simulink model "Manu6DOF_MICO_NE_v6articulation2019b"  (R2019b)
settings: Solver=ode5  StartTime=0.0  StopTime=10.0  FixedStep=0.001  RelTol=1e-3
undefined symbols (not defined in the file): f, Sub02MIHM
libraries: instrumentlib x27, dspnetwork x24, simulink x7, dspmtrx3 x3, dspsrcs4 x1
(part 1 of 3)
settings Model: Creator=nisit  LastModifiedBy=Jskyl

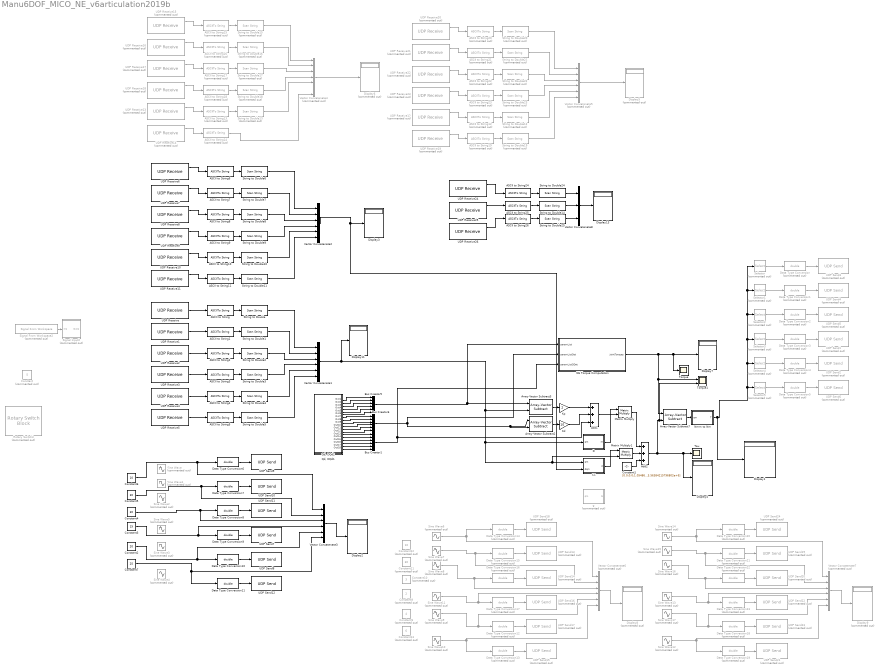
== system Manu6DOF_MICO_NE_v6articulation2019b ==
  ASCII to String{,1..11,24..26} (15 alike) : ASCIIToString
  ASCII to String{12..23} (12 alike) : ASCIIToString  Commented=on
  Add1 : Sum  Inputs=+++
  Add2 : Sum  Inputs=+++
  Array-Vector Subtract2 : dspmtrx3/Array-Vector Subtract  Dimension=1  V_Source=Input port  V_VectFromMask=[0.5 0.25]  prodOutputSignedness=Auto  roundingMode=Floor  overflowMode=off  firstCoeffSignedness=Auto  firstCoeffDataTypeStr=Inherit: Same word length as input  firstCoeffMin=[]  firstCoeffMax=[]  firstCoeffLastDataTypeStr=Inherit: Same word length as input  accumSignedness=Auto  outputSignedness=Auto  outputDataTypeStr=Inherit: Same as accumulator  outputMin=[]  outputMax=[]  outputLastDataTypeStr=Inherit: Same as accumulator
      settings: SourceProductBaseCode=DS
  Array-Vector Subtract3 : dspmtrx3/Array-Vector Subtract  Dimension=1  V_Source=Input port  V_VectFromMask=[0.5 0.25]  prodOutputSignedness=Auto  roundingMode=Floor  overflowMode=off  firstCoeffSignedness=Auto  firstCoeffDataTypeStr=Inherit: Same word length as input  firstCoeffMin=[]  firstCoeffMax=[]  firstCoeffLastDataTypeStr=Inherit: Same word length as input  accumSignedness=Auto  outputSignedness=Auto  outputDataTypeStr=Inherit: Same as accumulator  outputMin=[]  outputMax=[]  outputLastDataTypeStr=Inherit: Same as accumulator
      settings: SourceProductBaseCode=DS
  Array-Vector Subtract7 : dspmtrx3/Array-Vector Subtract  Dimension=1  V_Source=Input port  V_VectFromMask=[0.5 0.25]  prodOutputSignedness=Auto  roundingMode=Floor  overflowMode=off  firstCoeffSignedness=Auto  firstCoeffDataTypeStr=Inherit: Same word length as input  firstCoeffMin=[]  firstCoeffMax=[]  firstCoeffLastDataTypeStr=Inherit: Same word length as input  accumSignedness=Auto  outputSignedness=Auto  outputDataTypeStr=Inherit: Same as accumulator  outputMin=[]  outputMax=[]  outputLastDataTypeStr=Inherit: Same as accumulator
      settings: SourceProductBaseCode=DS
  Bus Creator1 : BusCreator  Inputs=6
  Bus Creator5 : BusCreator  Inputs=6
  Bus Creator6 : BusCreator  Inputs=6
  C1 : MATLAB Function  TreatAsAtomicUnit=on
  Constant : Constant  Commented=on  Value=5
  Constant1 : Constant  Value=[0.0;0.0;1.054861899110132e+7;sqrt(3.0).*2.596216141849145e-10+4.239942722516781e+6;sqrt(3.0).*2.389220043780056e-10-3.901892440242401e+6;sqrt(3.0).*(-6.546671837132898e-10)+3.56384215796802e+6]
  Constant10 : Constant  Commented=on  Value=3
  Constant11 : Constant  Commented=on  Value=30
  Constant12 : Constant  Commented=on  Value=10
  Constant13 : Constant  Commented=on  Value=6
  Constant2 : Constant  Value=20
  Constant3 : Constant  Value=15
  Constant4 : Constant  Value=30
  Constant5 : Constant  Value=30
  Constant6 : Constant  Value=10
  Constant7 : Constant  Value=25
  Constant8 : Constant  Commented=on  Value=4
  Constant9 : Constant  Commented=on  Value=2
  D : MATLAB Function  TreatAsAtomicUnit=on
  Data Type Conversion{,1..5,12..23} (18 alike) : DataTypeConversion  Commented=on  OutDataTypeStr=double  ConvertRealWorld=Stored Integer (SI)
  Data Type Conversion{6..11} (6 alike) : DataTypeConversion  OutDataTypeStr=double  ConvertRealWorld=Stored Integer (SI)
  Display{1..4,7,11,13} (7 alike) : Display
  Display{5..6,8..9} (4 alike) : Display  Commented=on
  Kd : Gain  Gain=10
  Kp : Gain  Gain=2
  Matrix Multiply : Product  Multiplication=Matrix(*)
  Matrix Multiply1 : Product  Multiplication=Matrix(*)
  NE Torque Computation : MATLAB Function  TreatAsAtomicUnit=on
  Nmm to Nm : MATLAB Function  TreatAsAtomicUnit=on
  "Qd, DQd1" : Subsystem
  "Qd, DQd2" : Subsystem
  Rotary Switch3 : RotarySwitchBlock  Commented=on
      settings: Values={{'Left', 'Right', 'Out', 'In', 'Up', 'Down'}, [1 4 2 5 3 6]}
  Selector : Selector  Commented=on  InputPortWidth=6  IndexOptions=Index vector (dialog)  Indices=[1]  OutputSizes=1
  Selector1 : Selector  Commented=on  InputPortWidth=6  IndexOptions=Index vector (dialog)  Indices=[2]  OutputSizes=1
  Selector2 : Selector  Commented=on  InputPortWidth=6  IndexOptions=Index vector (dialog)  Indices=[3]  OutputSizes=1
  Selector3 : Selector  Commented=on  InputPortWidth=6  IndexOptions=Index vector (dialog)  Indices=[4]  OutputSizes=1
  Selector4 : Selector  Commented=on  InputPortWidth=6  IndexOptions=Index vector (dialog)  Indices=[5]  OutputSizes=1
  Selector5 : Selector  Commented=on  InputPortWidth=6  IndexOptions=Index vector (dialog)  Indices=[6]  OutputSizes=1
  Signal From Workspace2 : dspsrcs4/Signal From Workspace  Commented=on  X=transpose(Sub02MIHM)  Ts=0.004  nsamps=1  OutputAfterFinalValue=Setting to zero  ignoreOrWarnInputAndFrameLengths=off  OutputFrames=off
  Signal Input2 : Subsystem  Commented=on
  Sine Wave : Sin  Commented=on  Amplitude=25  Frequency=15  SampleTime=0
  Sine Wave1 : Sin  Commented=on  Amplitude=30  Frequency=5  SampleTime=0
  Sine Wave10 : Sin  Commented=on  Amplitude=7  Frequency=8  SampleTime=0
  Sine Wave11 : Sin  Commented=on  Amplitude=9  Frequency=3  SampleTime=0
  Sine Wave12 : Sin  Commented=on  Amplitude=7  Frequency=8  SampleTime=0
  Sine Wave13 : Sin  Commented=on  Amplitude=9  Frequency=3  SampleTime=0
  Sine Wave14 : Sin  Commented=on  Amplitude=25  Frequency=15  SampleTime=0
  Sine Wave15 : Sin  Commented=on  Amplitude=30  Frequency=5  SampleTime=0
  Sine Wave16 : Sin  Commented=on  Amplitude=102  SampleTime=0
  Sine Wave17 : Sin  Commented=on  Amplitude=10  Frequency=15  SampleTime=0
  Sine Wave2 : Sin  Commented=on  Amplitude=102  SampleTime=0
  Sine Wave3 : Sin  Commented=on  Amplitude=10  Frequency=15  SampleTime=0
  Sine Wave4 : Sin  Commented=on  Amplitude=7  Frequency=8  SampleTime=0
  Sine Wave5 : Sin  Commented=on  Amplitude=9  Frequency=3  SampleTime=0
  Sine Wave6 : Sin  Commented=on  Amplitude=25  Frequency=15  SampleTime=0
  Sine Wave7 : Sin  Commented=on  Amplitude=30  Frequency=5  SampleTime=0
  Sine Wave8 : Sin  Commented=on  Amplitude=102  SampleTime=0
  Sine Wave9 : Sin  Commented=on  Amplitude=10  Frequency=15  SampleTime=0
  String to Double{,1..11,14,24..25} (15 alike) : ScanString  Format="\"%lf\""
  String to Double{12..13,15..23} (11 alike) : ScanString  Commented=on  Format="\"%lf\""
  Tau : Scope
  Torque : Scope
  Torque1 : Scope  NumInputPorts=2
  UDP Receive : instrumentlib/UDP Receive  Host=localhost  Port=2001  LocalPort=2001  EnablePortSharing=off  GetLatestData=off  DataSize="[5  1]"  DataType=uint8  ASCIIFormatting=%f,  Terminator=LF  ByteOrder=BigEndian  EnableBlockingMode=on  Timeout=10  SampleTime=0.01  LocalAddress=127.0.0.1
  UDP Receive1 : instrumentlib/UDP Receive  Host=localhost  Port=2002  LocalPort=2002  EnablePortSharing=off  GetLatestData=off  DataSize="[5  1]"  DataType=uint8  ASCIIFormatting=%f,  Terminator=LF  ByteOrder=BigEndian  EnableBlockingMode=on  Timeout=10  SampleTime=0.01  LocalAddress=127.0.0.1
  UDP Receive10 : instrumentlib/UDP Receive  Host=localhost  Port=4005  LocalPort=4005  EnablePortSharing=off  GetLatestData=off  DataSize="[5  1]"  DataType=uint8  ASCIIFormatting=%f,  Terminator=LF  ByteOrder=BigEndian  EnableBlockingMode=off  Timeout=10  SampleTime=0.01  LocalAddress=127.0.0.1
  UDP Receive11 : instrumentlib/UDP Receive  Host=localhost  Port=4006  LocalPort=4006  EnablePortSharing=off  GetLatestData=off  DataSize="[5  1]"  DataType=uint8  ASCIIFormatting=%f,  Terminator=LF  ByteOrder=BigEndian  EnableBlockingMode=off  Timeout=10  SampleTime=0.01  LocalAddress=127.0.0.1
  UDP Receive12 : instrumentlib/UDP Receive  Commented=on  Host=localhost  Port=7005  LocalPort=7005  EnablePortSharing=off  GetLatestData=off  DataSize="[5  1]"  DataType=uint8  ASCIIFormatting=%f,  Terminator=LF  ByteOrder=BigEndian  EnableBlockingMode=off  Timeout=10  SampleTime=0.01  LocalAddress=127.0.0.1
  UDP Receive13 : instrumentlib/UDP Receive  Commented=on  Host=localhost  Port=6005  LocalPort=6005  EnablePortSharing=off  GetLatestData=off  DataSize="[5  1]"  DataType=uint8  ASCIIFormatting=%f,  Terminator=LF  ByteOrder=BigEndian  EnableBlockingMode=off  Timeout=10  SampleTime=0.01  LocalAddress=127.0.0.1
  UDP Receive14 : instrumentlib/UDP Receive  Commented=on  Host=localhost  Port=6006  LocalPort=6006  EnablePortSharing=off  GetLatestData=off  DataSize="[5  1]"  DataType=uint8  ASCIIFormatting=%f,  Terminator=LF  ByteOrder=BigEndian  EnableBlockingMode=off  Timeout=10  SampleTime=0.01  LocalAddress=127.0.0.1
  UDP Receive15 : instrumentlib/UDP Receive  Commented=on  Host=localhost  Port=6001  LocalPort=6001  EnablePortSharing=off  GetLatestData=off  DataSize="[5  1]"  DataType=uint8  ASCIIFormatting=%f,  Terminator=LF  ByteOrder=BigEndian  EnableBlockingMode=off  Timeout=10  SampleTime=0.01  LocalAddress=127.0.0.1
  UDP Receive16 : instrumentlib/UDP Receive  Commented=on  Host=localhost  Port=6002  LocalPort=6002  EnablePortSharing=off  GetLatestData=off  DataSize="[5  1]"  DataType=uint8  ASCIIFormatting=%f,  Terminator=LF  ByteOrder=BigEndian  EnableBlockingMode=off  Timeout=10  SampleTime=0.01  LocalAddress=127.0.0.1
  UDP Receive17 : instrumentlib/UDP Receive  Commented=on  Host=localhost  Port=6003  LocalPort=6003  EnablePortSharing=off  GetLatestData=off  DataSize="[5  1]"  DataType=uint8  ASCIIFormatting=%f,  Terminator=LF  ByteOrder=BigEndian  EnableBlockingMode=off  Timeout=10  SampleTime=0.01  LocalAddress=127.0.0.1
  UDP Receive18 : instrumentlib/UDP Receive  Commented=on  Host=localhost  Port=6004  LocalPort=6004  EnablePortSharing=off  GetLatestData=off  DataSize="[5  1]"  DataType=uint8  ASCIIFormatting=%f,  Terminator=LF  ByteOrder=BigEndian  EnableBlockingMode=off  Timeout=10  SampleTime=0.01  LocalAddress=127.0.0.1
  UDP Receive19 : instrumentlib/UDP Receive  Commented=on  Host=localhost  Port=7006  LocalPort=7006  EnablePortSharing=off  GetLatestData=off  DataSize="[5  1]"  DataType=uint8  ASCIIFormatting=%f,  Terminator=LF  ByteOrder=BigEndian  EnableBlockingMode=off  Timeout=10  SampleTime=0.01  LocalAddress=127.0.0.1
  UDP Receive2 : instrumentlib/UDP Receive  Host=localhost  Port=2003  LocalPort=2003  EnablePortSharing=off  GetLatestData=off  DataSize="[5  1]"  DataType=uint8  ASCIIFormatting=%f,  Terminator=LF  ByteOrder=BigEndian  EnableBlockingMode=on  Timeout=10  SampleTime=0.01  LocalAddress=127.0.0.1
  UDP Receive20 : instrumentlib/UDP Receive  Commented=on  Host=localhost  Port=7001  LocalPort=7001  EnablePortSharing=off  GetLatestData=off  DataSize="[5  1]"  DataType=uint8  ASCIIFormatting=%f,  Terminator=LF  ByteOrder=BigEndian  EnableBlockingMode=off  Timeout=10  SampleTime=0.01  LocalAddress=127.0.0.1
  UDP Receive21 : instrumentlib/UDP Receive  Commented=on  Host=localhost  Port=7002  LocalPort=7002  EnablePortSharing=off  GetLatestData=off  DataSize="[5  1]"  DataType=uint8  ASCIIFormatting=%f,  Terminator=LF  ByteOrder=BigEndian  EnableBlockingMode=off  Timeout=10  SampleTime=0.01  LocalAddress=127.0.0.1
  UDP Receive22 : instrumentlib/UDP Receive  Commented=on  Host=localhost  Port=7003  LocalPort=7003  EnablePortSharing=off  GetLatestData=off  DataSize="[5  1]"  DataType=uint8  ASCIIFormatting=%f,  Terminator=LF  ByteOrder=BigEndian  EnableBlockingMode=off  Timeout=10  SampleTime=0.01  LocalAddress=127.0.0.1
  UDP Receive23 : instrumentlib/UDP Receive  Commented=on  Host=localhost  Port=7004  LocalPort=7004  EnablePortSharing=off  GetLatestData=off  DataSize="[5  1]"  DataType=uint8  ASCIIFormatting=%f,  Terminator=LF  ByteOrder=BigEndian  EnableBlockingMode=off  Timeout=10  SampleTime=0.01  LocalAddress=127.0.0.1
  UDP Receive24 : instrumentlib/UDP Receive  Host=localhost  Port=5100  LocalPort=5100  EnablePortSharing=off  GetLatestData=off  DataSize="[5  1]"  DataType=uint8  ASCIIFormatting=%f,  Terminator=LF  ByteOrder=BigEndian  EnableBlockingMode=off  Timeout=10  SampleTime=0.01  LocalAddress=127.0.0.1
  UDP Receive25 : instrumentlib/UDP Receive  Host=localhost  Port=5200  LocalPort=5200  EnablePortSharing=off  GetLatestData=off  DataSize="[5  1]"  DataType=uint8  ASCIIFormatting=%f,  Terminator=LF  ByteOrder=BigEndian  EnableBlockingMode=off  Timeout=10  SampleTime=0.01  LocalAddress=127.0.0.1
  UDP Receive26 : instrumentlib/UDP Receive  Host=localhost  Port=5300  LocalPort=5300  EnablePortSharing=off  GetLatestData=off  DataSize="[5  1]"  DataType=uint8  ASCIIFormatting=%f,  Terminator=LF  ByteOrder=BigEndian  EnableBlockingMode=off  Timeout=10  SampleTime=0.01  LocalAddress=127.0.0.1
  UDP Receive3 : instrumentlib/UDP Receive  Host=localhost  Port=2004  LocalPort=2004  EnablePortSharing=off  GetLatestData=off  DataSize="[5  1]"  DataType=uint8  ASCIIFormatting=%f,  Terminator=LF  ByteOrder=BigEndian  EnableBlockingMode=on  Timeout=10  SampleTime=0.01  LocalAddress=127.0.0.1
  UDP Receive4 : instrumentlib/UDP Receive  Host=localhost  Port=2005  LocalPort=2005  EnablePortSharing=off  GetLatestData=off  DataSize="[5  1]"  DataType=uint8  ASCIIFormatting=%f,  Terminator=LF  ByteOrder=BigEndian  EnableBlockingMode=on  Timeout=10  SampleTime=0.01  LocalAddress=127.0.0.1
  UDP Receive5 : instrumentlib/UDP Receive  Host=localhost  Port=2006  LocalPort=2006  EnablePortSharing=off  GetLatestData=off  DataSize="[5  1]"  DataType=uint8  ASCIIFormatting=%f,  Terminator=LF  ByteOrder=BigEndian  EnableBlockingMode=on  Timeout=10  SampleTime=0.01  LocalAddress=127.0.0.1
  UDP Receive6 : instrumentlib/UDP Receive  Host=localhost  Port=4001  LocalPort=4001  EnablePortSharing=off  GetLatestData=off  DataSize="[5  1]"  DataType=uint8  ASCIIFormatting=%f,  Terminator=LF  ByteOrder=BigEndian  EnableBlockingMode=off  Timeout=10  SampleTime=0.01  LocalAddress=127.0.0.1
  UDP Receive7 : instrumentlib/UDP Receive  Host=localhost  Port=4002  LocalPort=4002  EnablePortSharing=off  GetLatestData=off  DataSize="[5  1]"  DataType=uint8  ASCIIFormatting=%f,  Terminator=LF  ByteOrder=BigEndian  EnableBlockingMode=off  Timeout=10  SampleTime=0.01  LocalAddress=127.0.0.1
  UDP Receive8 : instrumentlib/UDP Receive  Host=localhost  Port=4003  LocalPort=4003  EnablePortSharing=off  GetLatestData=off  DataSize="[5  1]"  DataType=uint8  ASCIIFormatting=%f,  Terminator=LF  ByteOrder=BigEndian  EnableBlockingMode=off  Timeout=10  SampleTime=0.01  LocalAddress=127.0.0.1
  UDP Receive9 : instrumentlib/UDP Receive  Host=localhost  Port=4004  LocalPort=4004  EnablePortSharing=off  GetLatestData=off  DataSize="[5  1]"  DataType=uint8  ASCIIFormatting=%f,  Terminator=LF  ByteOrder=BigEndian  EnableBlockingMode=off  Timeout=10  SampleTime=0.01  LocalAddress=127.0.0.1
  UDP Send1 : dspnetwork/UDP Send  Commented=on  remoteURL='127.0.0.1'  remotePort=3004  localURL='0.0.0.0'  localPortSource=Automatically determine  localPort=-1  sampletime=-1  blockPlatform=[]  separateLengthPort=0
  UDP Send10 : dspnetwork/UDP Send  remoteURL='127.0.0.1'  remotePort=5002  localURL='0.0.0.0'  localPortSource=Automatically determine  localPort=-1  sampletime=-1  blockPlatform=[]  separateLengthPort=0
  UDP Send11 : dspnetwork/UDP Send  remoteURL='127.0.0.1'  remotePort=5003  localURL='0.0.0.0'  localPortSource=Automatically determine  localPort=-1  sampletime=-1  blockPlatform=[]  separateLengthPort=0
  UDP Send12 : dspnetwork/UDP Send  remoteURL='127.0.0.1'  remotePort=5006  localURL='0.0.0.0'  localPortSource=Automatically determine  localPort=-1  sampletime=-1  blockPlatform=[]  separateLengthPort=0
  UDP Send13 : dspnetwork/UDP Send  Commented=on  remoteURL='127.0.0.1'  remotePort=8002  localURL='0.0.0.0'  localPortSource=Automatically determine  localPort=-1  sampletime=-1  blockPlatform=[]  separateLengthPort=0
  UDP Send14 : dspnetwork/UDP Send  Commented=on  remoteURL='127.0.0.1'  remotePort=8003  localURL='0.0.0.0'  localPortSource=Automatically determine  localPort=-1  sampletime=-1  blockPlatform=[]  separateLengthPort=0
  UDP Send15 : dspnetwork/UDP Send  Commented=on  remoteURL='127.0.0.1'  remotePort=8006  localURL='0.0.0.0'  localPortSource=Automatically determine  localPort=-1  sampletime=-1  blockPlatform=[]  separateLengthPort=0
  UDP Send16 : dspnetwork/UDP Send  Commented=on  remoteURL='127.0.0.1'  remotePort=8004  localURL='0.0.0.0'  localPortSource=Automatically determine  localPort=-1  sampletime=-1  blockPlatform=[]  separateLengthPort=0
  UDP Send17 : dspnetwork/UDP Send  Commented=on  remoteURL='127.0.0.1'  remotePort=8005  localURL='0.0.0.0'  localPortSource=Automatically determine  localPort=-1  sampletime=-1  blockPlatform=[]  separateLengthPort=0
  UDP Send18 : dspnetwork/UDP Send  Commented=on  remoteURL='127.0.0.1'  remotePort=8001  localURL='0.0.0.0'  localPortSource=Automatically determine  localPort=-1  sampletime=-1  blockPlatform=[]  separateLengthPort=0
  UDP Send19 : dspnetwork/UDP Send  Commented=on  remoteURL='127.0.0.1'  remotePort=9002  localURL='0.0.0.0'  localPortSource=Automatically determine  localPort=-1  sampletime=-1  blockPlatform=[]  separateLengthPort=0
  UDP Send2 : dspnetwork/UDP Send  Commented=on  remoteURL='127.0.0.1'  remotePort=3005  localURL='0.0.0.0'  localPortSource=Automatically determine  localPort=-1  sampletime=-1  blockPlatform=[]  separateLengthPort=0
  UDP Send20 : dspnetwork/UDP Send  Commented=on  remoteURL='127.0.0.1'  remotePort=9003  localURL='0.0.0.0'  localPortSource=Automatically determine  localPort=-1  sampletime=-1  blockPlatform=[]  separateLengthPort=0
  UDP Send21 : dspnetwork/UDP Send  Commented=on  remoteURL='127.0.0.1'  remotePort=9006  localURL='0.0.0.0'  localPortSource=Automatically determine  localPort=-1  sampletime=-1  blockPlatform=[]  separateLengthPort=0
  UDP Send22 : dspnetwork/UDP Send  Commented=on  remoteURL='127.0.0.1'  remotePort=9004  localURL='0.0.0.0'  localPortSource=Automatically determine  localPort=-1  sampletime=-1  blockPlatform=[]  separateLengthPort=0
  UDP Send23 : dspnetwork/UDP Send  Commented=on  remoteURL='127.0.0.1'  remotePort=9005  localURL='0.0.0.0'  localPortSource=Automatically determine  localPort=-1  sampletime=-1  blockPlatform=[]  separateLengthPort=0
  UDP Send24 : dspnetwork/UDP Send  Commented=on  remoteURL='127.0.0.1'  remotePort=9001  localURL='0.0.0.0'  localPortSource=Automatically determine  localPort=-1  sampletime=-1  blockPlatform=[]  separateLengthPort=0
  UDP Send3 : dspnetwork/UDP Send  Commented=on  remoteURL='127.0.0.1'  remotePort=3001  localURL='0.0.0.0'  localPortSource=Automatically determine  localPort=-1  sampletime=-1  blockPlatform=[]  separateLengthPort=0
  UDP Send4 : dspnetwork/UDP Send  Commented=on  remoteURL='127.0.0.1'  remotePort=3002  localURL='0.0.0.0'  localPortSource=Automatically determine  localPort=-1  sampletime=-1  blockPlatform=[]  separateLengthPort=0
  UDP Send5 : dspnetwork/UDP Send  Commented=on  remoteURL='127.0.0.1'  remotePort=3003  localURL='0.0.0.0'  localPortSource=Automatically determine  localPort=-1  sampletime=-1  blockPlatform=[]  separateLengthPort=0
  UDP Send6 : dspnetwork/UDP Send  Commented=on  remoteURL='127.0.0.1'  remotePort=3006  localURL='0.0.0.0'  localPortSource=Automatically determine  localPort=-1  sampletime=-1  blockPlatform=[]  separateLengthPort=0
  UDP Send7 : dspnetwork/UDP Send  remoteURL='127.0.0.1'  remotePort=5004  localURL='0.0.0.0'  localPortSource=Automatically determine  localPort=-1  sampletime=-1  blockPlatform=[]  separateLengthPort=0
  UDP Send8 : dspnetwork/UDP Send  remoteURL='127.0.0.1'  remotePort=5005  localURL='0.0.0.0'  localPortSource=Automatically determine  localPort=-1  sampletime=-1  blockPlatform=[]  separateLengthPort=0
  UDP Send9 : dspnetwork/UDP Send  remoteURL='127.0.0.1'  remotePort=5001  localURL='0.0.0.0'  localPortSource=Automatically determine  localPort=-1  sampletime=-1  blockPlatform=[]  separateLengthPort=0
  Vector Concatenate1 : Concatenate  NumInputs=6
  Vector Concatenate2 : Concatenate  NumInputs=6
  Vector Concatenate3 : Concatenate  NumInputs=6
  Vector Concatenate4 : Concatenate  Commented=on  NumInputs=7
  Vector Concatenate5 : Concatenate  Commented=on  NumInputs=6
  Vector Concatenate6 : Concatenate  Commented=on  NumInputs=6
  Vector Concatenate7 : Concatenate  Commented=on  NumInputs=6
  Vector Concatenate8 : Concatenate  NumInputs=3
  g : MATLAB Function  Commented=on  TreatAsAtomicUnit=on
  wires:
  D/1(M) -> Matrix Multiply/1
  Matrix Multiply1/1 -> Add2/2
  Array-Vector Subtract3/1 -> Kp/1
  Array-Vector Subtract2/1 -> Kd/1
  Matrix Multiply/1 -> Add2/1
  Kd/1 -> Add1/2
  Add1/1 -> Matrix Multiply/2
  Kp/1 -> Add1/1
  C1/1(C) -> Matrix Multiply1/1
  Array-Vector Subtract7/1 -> Nmm to Nm/1(qm)
  Add2/1 -> Torque1/2, Array-Vector Subtract7/2, Display4/1, Tau/1
  Constant1/1 -> Add2/3
  "Qd, DQd1"/15(Out15) -> Bus Creator1/3
  "Qd, DQd1"/10(Out10) -> Bus Creator6/4
  "Qd, DQd1"/17(Out17) -> Bus Creator1/5
  "Qd, DQd1"/9(Out9) -> Bus Creator6/3
  "Qd, DQd1"/11(Out11) -> Bus Creator6/5
  "Qd, DQd1"/6(Out6) -> Bus Creator5/6
  "Qd, DQd1"/12(Out12) -> Bus Creator6/6
  "Qd, DQd1"/13(Out13) -> Bus Creator1/1
  "Qd, DQd1"/18(Out18) -> Bus Creator1/6
  "Qd, DQd1"/16(Out16) -> Bus Creator1/4
  "Qd, DQd1"/1(Out1) -> Bus Creator5/1
  "Qd, DQd1"/2(Out2) -> Bus Creator5/2
  "Qd, DQd1"/7(Out7) -> Bus Creator6/1
  "Qd, DQd1"/5(Out5) -> Bus Creator5/5
  "Qd, DQd1"/3(Out3) -> Bus Creator5/3
  "Qd, DQd1"/8(Out8) -> Bus Creator6/2
  "Qd, DQd1"/14(Out14) -> Bus Creator1/2
  "Qd, DQd1"/4(Out4) -> Bus Creator5/4
  Signal From Workspace2/1 -> Signal Input2/1(In1)
  Data Type Conversion2/1 -> UDP Send5/1
  Selector5/1 -> Data Type Conversion5/1
  Data Type Conversion5/1 -> UDP Send6/1
  Selector4/1 -> Data Type Conversion4/1
  Data Type Conversion3/1 -> UDP Send1/1
  Data Type Conversion1/1 -> UDP Send4/1
  Data Type Conversion4/1 -> UDP Send2/1
  Selector2/1 -> Data Type Conversion2/1
  Selector/1 -> Data Type Conversion/1
  Selector1/1 -> Data Type Conversion1/1
  Data Type Conversion/1 -> UDP Send3/1
  Selector3/1 -> Data Type Conversion3/1
  NE Torque Computation/1(jointTorques) -> Display7/1, Torque/1, Array-Vector Subtract7/1, Torque1/1
  String to Double4/1 -> Vector Concatenate1/5
  ASCII to String2/1 -> String to Double2/1
  String to Double/1 -> Vector Concatenate1/1
  ASCII to String4/1 -> String to Double4/1
  String to Double2/1 -> Vector Concatenate1/3
  ASCII to String3/1 -> String to Double3/1
  String to Double5/1 -> Vector Concatenate1/6
  String to Double1/1 -> Vector Concatenate1/2
  ASCII to String1/1 -> String to Double1/1
  UDP Receive2/1 -> ASCII to String2/1
  UDP Receive/1 -> ASCII to String/1
  ASCII to String5/1 -> String to Double5/1
  UDP Receive3/1 -> ASCII to String3/1
  UDP Receive1/1 -> ASCII to String1/1
  ASCII to String/1 -> String to Double/1
  UDP Receive5/1 -> ASCII to String5/1
  UDP Receive4/1 -> ASCII to String4/1
  String to Double3/1 -> Vector Concatenate1/4
  Bus Creator6/1 -> NE Torque Computation/2(paramListDot), Array-Vector Subtract2/2, Array-Vector Subtract2/1
  Vector Concatenate1/1 -> Display11/1, Matrix Multiply1/2, C1/1(qm), D/1(qm), Array-Vector Subtract3/2
  Bus Creator5/1 -> Array-Vector Subtract3/1, NE Torque Computation/1(paramList)
  Bus Creator1/1 -> Add1/3, NE Torque Computation/3(paramListDDot)
  Nmm to Nm/1(T) -> Display1/1, Selector/1, Selector1/1, Selector2/1, Selector3/1, Selector4/1, Selector5/1
  Data Type Conversion6/1 -> UDP Send9/1
  Data Type Conversion7/1 -> UDP Send10/1
  Data Type Conversion8/1 -> UDP Send11/1
  Data Type Conversion11/1 -> UDP Send12/1
  Data Type Conversion10/1 -> UDP Send8/1
  Data Type Conversion9/1 -> UDP Send7/1
  ASCII to String7/1 -> String to Double7/1
  UDP Receive6/1 -> ASCII to String6/1
  UDP Receive9/1 -> ASCII to String9/1
  String to Double6/1 -> Vector Concatenate2/1
  ASCII to String11/1 -> String to Double11/1
  String to Double8/1 -> Vector Concatenate2/3
  ASCII to String9/1 -> String to Double9/1
  String to Double11/1 -> Vector Concatenate2/6
  UDP Receive10/1 -> ASCII to String10/1
  UDP Receive8/1 -> ASCII to String8/1
  String to Double10/1 -> Vector Concatenate2/5
  UDP Receive7/1 -> ASCII to String7/1
  ASCII to String10/1 -> String to Double10/1
  String to Double9/1 -> Vector Concatenate2/4
  UDP Receive11/1 -> ASCII to String11/1
  ASCII to String8/1 -> String to Double8/1
  String to Double7/1 -> Vector Concatenate2/2
  ASCII to String6/1 -> String to Double6/1
  Vector Concatenate2/1 -> C1/2(dqm), Display3/1
  Vector Concatenate3/1 -> Display2/1
  Constant2/1 -> Vector Concatenate3/5, Data Type Conversion10/1
  Constant3/1 -> Vector Concatenate3/4, Data Type Conversion9/1
  Constant4/1 -> Vector Concatenate3/3, Data Type Conversion8/1
  Constant5/1 -> Vector Concatenate3/2, Data Type Conversion7/1
  Constant6/1 -> Vector Concatenate3/1, Data Type Conversion6/1
  Constant7/1 -> Vector Concatenate3/6, Data Type Conversion11/1
  String to Double13/1 -> Vector Concatenate4/5
  UDP Receive15/1 -> ASCII to String15/1
  Vector Concatenate4/1 -> Display6/1
  ASCII to String16/1 -> String to Double16/1
  String to Double18/1 -> Vector Concatenate4/4
  UDP Receive17/1 -> ASCII to String17/1
  UDP Receive16/1 -> ASCII to String16/1
  ASCII to String15/1 -> String to Double15/1
  UDP Receive14/1 -> ASCII to String14/1
  ASCII to String13/1 -> String to Double13/1
  UDP Receive13/1 -> ASCII to String13/1
  ASCII to String18/1 -> String to Double18/1
  ASCII to String17/1 -> String to Double17/1
  String to Double15/1 -> Vector Concatenate4/1
  UDP Receive18/1 -> ASCII to String18/1
  String to Double16/1 -> Vector Concatenate4/2
  String to Double17/1 -> Vector Concatenate4/3
  String to Double12/1 -> Vector Concatenate5/5
  UDP Receive20/1 -> ASCII to String20/1
  Vector Concatenate5/1 -> Display5/1
  ASCII to String21/1 -> String to Double21/1
  String to Double23/1 -> Vector Concatenate5/4
  ASCII to String19/1 -> String to Double19/1
  UDP Receive22/1 -> ASCII to String22/1
  String to Double19/1 -> Vector Concatenate5/6
  UDP Receive21/1 -> ASCII to String21/1
  ASCII to String20/1 -> String to Double20/1
  UDP Receive19/1 -> ASCII to String19/1
  ASCII to String12/1 -> String to Double12/1
  UDP Receive12/1 -> ASCII to String12/1
  ASCII to String23/1 -> String to Double23/1
  ASCII to String22/1 -> String to Double22/1
  String to Double20/1 -> Vector Concatenate5/1
  UDP Receive23/1 -> ASCII to String23/1
  String to Double21/1 -> Vector Concatenate5/2
  String to Double22/1 -> Vector Concatenate5/3
  Vector Concatenate6/1 -> Display8/1
  Data Type Conversion15/1 -> UDP Send13/1
  Data Type Conversion12/1 -> UDP Send17/1
  Data Type Conversion13/1 -> UDP Send15/1
  Data Type Conversion14/1 -> UDP Send18/1
  Data Type Conversion17/1 -> UDP Send16/1
  Data Type Conversion16/1 -> UDP Send14/1
  Sine Wave6/1 -> Vector Concatenate6/1, Data Type Conversion14/1
  Sine Wave7/1 -> Vector Concatenate6/2, Data Type Conversion15/1
  Sine Wave8/1 -> Vector Concatenate6/3, Data Type Conversion16/1
  Sine Wave11/1 -> Vector Concatenate6/4, Data Type Conversion17/1
  Sine Wave9/1 -> Vector Concatenate6/5, Data Type Conversion12/1
  Sine Wave10/1 -> Data Type Conversion13/1, Vector Concatenate6/6
  Sine Wave15/1 -> Vector Concatenate7/2, Data Type Conversion21/1
  Data Type Conversion20/1 -> UDP Send24/1
  Data Type Conversion19/1 -> UDP Send21/1
  Data Type Conversion18/1 -> UDP Send23/1
  Sine Wave12/1 -> Data Type Conversion19/1, Vector Concatenate7/6
  Data Type Conversion21/1 -> UDP Send19/1
  Data Type Conversion23/1 -> UDP Send22/1
  Vector Concatenate7/1 -> Display9/1
  Sine Wave17/1 -> Vector Concatenate7/5, Data Type Conversion18/1
  Sine Wave14/1 -> Vector Concatenate7/1, Data Type Conversion20/1
  Sine Wave16/1 -> Vector Concatenate7/3, Data Type Conversion22/1
  Data Type Conversion22/1 -> UDP Send20/1
  Sine Wave13/1 -> Vector Concatenate7/4, Data Type Conversion23/1
  UDP Receive24/1 -> ASCII to String24/1
  ASCII to String24/1 -> String to Double24/1
  String to Double24/1 -> Vector Concatenate8/1
  ASCII to String14/1 -> Vector Concatenate4/7
  ASCII to String25/1 -> String to Double14/1
  String to Double14/1 -> Vector Concatenate8/2
  UDP Receive25/1 -> ASCII to String25/1
  ASCII to String26/1 -> String to Double25/1
  UDP Receive26/1 -> ASCII to String26/1
  String to Double25/1 -> Vector Concatenate8/3
  Vector Concatenate8/1 -> Display13/1

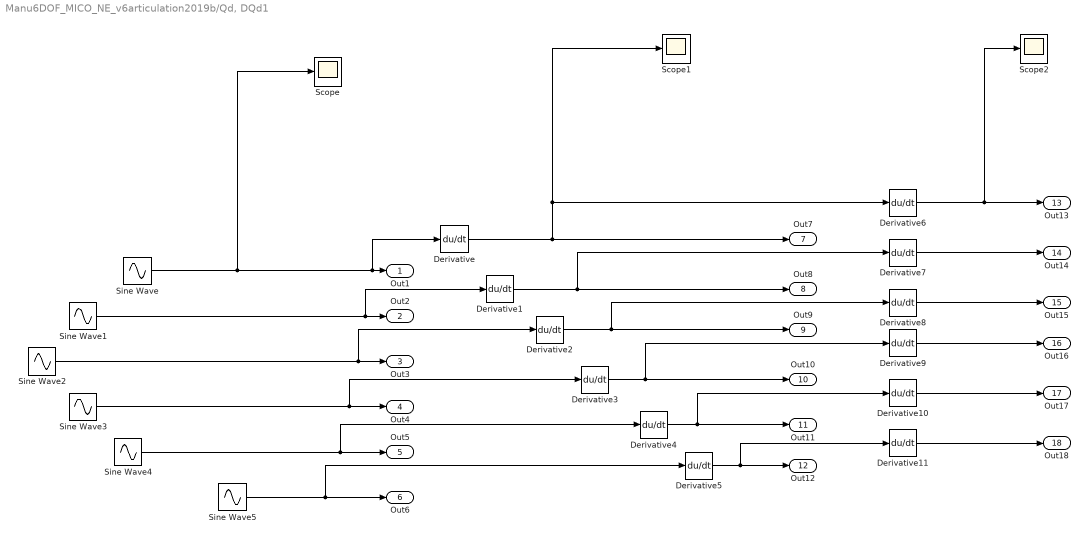
== system Manu6DOF_MICO_NE_v6articulation2019b/Qd, DQd1 ==
  Derivative{,1..11} (12 alike) : Derivative
  Scope : Scope
  Scope1 : Scope
  Scope2 : Scope
  Sine Wave : Sin  Amplitude=.1  SampleTime=0
  Sine Wave{1..5} (5 alike) : Sin  SampleTime=0
  Out1 : Outport  VectorParamsAs1DForOutWhenUnconnected=off
  Out2 : Outport  Port=2  VectorParamsAs1DForOutWhenUnconnected=off
  Out3 : Outport  Port=3  VectorParamsAs1DForOutWhenUnconnected=off
  Out4 : Outport  Port=4  VectorParamsAs1DForOutWhenUnconnected=off
  Out5 : Outport  Port=5  VectorParamsAs1DForOutWhenUnconnected=off
  Out6 : Outport  Port=6  VectorParamsAs1DForOutWhenUnconnected=off
  Out7 : Outport  Port=7  VectorParamsAs1DForOutWhenUnconnected=off
  Out8 : Outport  Port=8  VectorParamsAs1DForOutWhenUnconnected=off
  Out9 : Outport  Port=9  VectorParamsAs1DForOutWhenUnconnected=off
  Out10 : Outport  Port=10  VectorParamsAs1DForOutWhenUnconnected=off
  Out11 : Outport  Port=11  VectorParamsAs1DForOutWhenUnconnected=off
  Out12 : Outport  Port=12  VectorParamsAs1DForOutWhenUnconnected=off
  Out13 : Outport  Port=13  VectorParamsAs1DForOutWhenUnconnected=off
  Out14 : Outport  Port=14  VectorParamsAs1DForOutWhenUnconnected=off
  Out15 : Outport  Port=15  VectorParamsAs1DForOutWhenUnconnected=off
  Out16 : Outport  Port=16  VectorParamsAs1DForOutWhenUnconnected=off
  Out17 : Outport  Port=17  VectorParamsAs1DForOutWhenUnconnected=off
  Out18 : Outport  Port=18  VectorParamsAs1DForOutWhenUnconnected=off
  wires:
  Derivative11/1 -> Out18/1
  Derivative10/1 -> Out17/1
  Derivative9/1 -> Out16/1
  Derivative8/1 -> Out15/1
  Derivative7/1 -> Out14/1
  Derivative6/1 -> Out13/1, Scope2/1
  Derivative1/1 -> Out8/1, Derivative7/1
  Derivative/1 -> Out7/1, Derivative6/1, Scope1/1
  Derivative2/1 -> Out9/1, Derivative8/1
  Derivative3/1 -> Out10/1, Derivative9/1
  Derivative4/1 -> Out11/1, Derivative10/1
  Derivative5/1 -> Out12/1, Derivative11/1
  Sine Wave5/1 -> Out6/1, Derivative5/1
  Sine Wave4/1 -> Out5/1, Derivative4/1
  Sine Wave3/1 -> Out4/1, Derivative3/1
  Sine Wave2/1 -> Out3/1, Derivative2/1
  Sine Wave1/1 -> Out2/1, Derivative1/1
  Sine Wave/1 -> Out1/1, Derivative/1, Scope/1

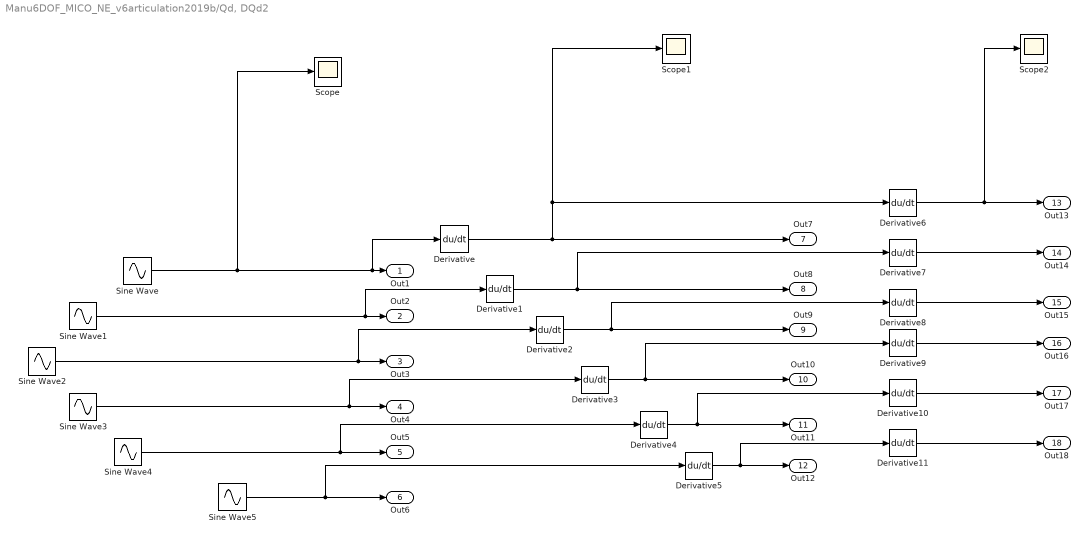
== system Manu6DOF_MICO_NE_v6articulation2019b/Qd, DQd2 ==
  Derivative{,1..11} (12 alike) : Derivative
  Scope : Scope
  Scope1 : Scope
  Scope2 : Scope
  Sine Wave : Sin  Amplitude=.1  SampleTime=0
  Sine Wave{1..5} (5 alike) : Sin  SampleTime=0
  Out1 : Outport  VectorParamsAs1DForOutWhenUnconnected=off
  Out2 : Outport  Port=2  VectorParamsAs1DForOutWhenUnconnected=off
  Out3 : Outport  Port=3  VectorParamsAs1DForOutWhenUnconnected=off
  Out4 : Outport  Port=4  VectorParamsAs1DForOutWhenUnconnected=off
  Out5 : Outport  Port=5  VectorParamsAs1DForOutWhenUnconnected=off
  Out6 : Outport  Port=6  VectorParamsAs1DForOutWhenUnconnected=off
  Out7 : Outport  Port=7  VectorParamsAs1DForOutWhenUnconnected=off
  Out8 : Outport  Port=8  VectorParamsAs1DForOutWhenUnconnected=off
  Out9 : Outport  Port=9  VectorParamsAs1DForOutWhenUnconnected=off
  Out10 : Outport  Port=10  VectorParamsAs1DForOutWhenUnconnected=off
  Out11 : Outport  Port=11  VectorParamsAs1DForOutWhenUnconnected=off
  Out12 : Outport  Port=12  VectorParamsAs1DForOutWhenUnconnected=off
  Out13 : Outport  Port=13  VectorParamsAs1DForOutWhenUnconnected=off
  Out14 : Outport  Port=14  VectorParamsAs1DForOutWhenUnconnected=off
  Out15 : Outport  Port=15  VectorParamsAs1DForOutWhenUnconnected=off
  Out16 : Outport  Port=16  VectorParamsAs1DForOutWhenUnconnected=off
  Out17 : Outport  Port=17  VectorParamsAs1DForOutWhenUnconnected=off
  Out18 : Outport  Port=18  VectorParamsAs1DForOutWhenUnconnected=off
  wires:
  Sine Wave/1 -> Scope/1, Derivative/1, Out1/1
  Sine Wave1/1 -> Derivative1/1, Out2/1
  Sine Wave2/1 -> Derivative2/1, Out3/1
  Sine Wave3/1 -> Derivative3/1, Out4/1
  Sine Wave4/1 -> Derivative4/1, Out5/1
  Sine Wave5/1 -> Derivative5/1, Out6/1
  Derivative5/1 -> Derivative11/1, Out12/1
  Derivative4/1 -> Derivative10/1, Out11/1
  Derivative3/1 -> Derivative9/1, Out10/1
  Derivative2/1 -> Derivative8/1, Out9/1
  Derivative/1 -> Scope1/1, Derivative6/1, Out7/1
  Derivative1/1 -> Derivative7/1, Out8/1
  Derivative6/1 -> Scope2/1, Out13/1
  Derivative7/1 -> Out14/1
  Derivative8/1 -> Out15/1
  Derivative9/1 -> Out16/1
  Derivative10/1 -> Out17/1
  Derivative11/1 -> Out18/1

== system Manu6DOF_MICO_NE_v6articulation2019b/Signal Input2 ==
  In1 : Inport
  Iterator Input : Subsystem
  Subsystem1 : Subsystem
  Out1 : Outport
  wires:
  Subsystem1/1(Out1) -> Iterator Input/1(In1)
  Subsystem1/3(Out3) -> Iterator Input/3(In3)
  In1/1 -> Subsystem1/1(In1)
  Subsystem1/4(Out4) -> Iterator Input/4(In4)
  Subsystem1/7(Out7) -> Iterator Input/7(In7)
  Subsystem1/2(Out2) -> Iterator Input/2(In2)
  Subsystem1/6(Out6) -> Iterator Input/6(In6)
  Subsystem1/5(Out5) -> Iterator Input/5(In5)
  Iterator Input/1(Out1) -> Out1/1

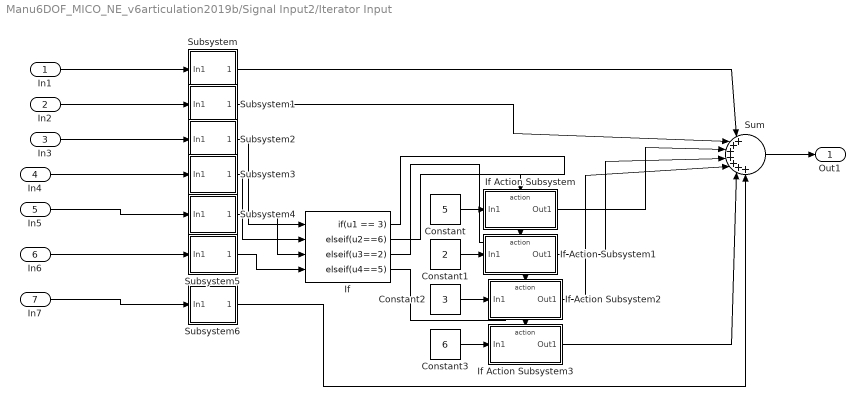
== system Manu6DOF_MICO_NE_v6articulation2019b/Signal Input2/Iterator Input ==
  In1 : Inport
  In2 : Inport  Port=2
  In3 : Inport  Port=3
  In4 : Inport  Port=4
  In5 : Inport  Port=5
  In6 : Inport  Port=6
  In7 : Inport  Port=7
  Constant : Constant  Value=5
  Constant1 : Constant  Value=2
  Constant2 : Constant  Value=3
  Constant3 : Constant  Value=6
  If : If  NumInputs=4  IfExpression=u1 == 3  ElseIfExpressions=u2==6,u3==2,u4==5  ShowElse=off
  If Action Subsystem : Subsystem  TreatAsAtomicUnit=on
  If Action Subsystem1 : Subsystem  TreatAsAtomicUnit=on
  If Action Subsystem2 : Subsystem  TreatAsAtomicUnit=on
  If Action Subsystem3 : Subsystem  TreatAsAtomicUnit=on
  Subsystem : Subsystem
  Subsystem1 : Subsystem
  Subsystem2 : Subsystem
  Subsystem3 : Subsystem
  Subsystem4 : Subsystem
  Subsystem5 : Subsystem
  Subsystem6 : Subsystem
  Sum : Sum  Inputs=|+++++++
  Out1 : Outport
  wires:
  Sum/1 -> Out1/1
  In5/1 -> Subsystem4/1(In1)
  In2/1 -> Subsystem1/1(In1)
  Subsystem/1(Out1) -> Sum/1
  In4/1 -> Subsystem3/1(In1)
  Subsystem1/1(Out1) -> Sum/2
  In1/1 -> Subsystem/1(In1)
  In3/1 -> Subsystem2/1(In1)
  In6/1 -> Subsystem5/1(In1)
  In7/1 -> Subsystem6/1(In1)
  If/1 -> If Action Subsystem/Action
  Constant/1 -> If Action Subsystem/1(In1)
  If/2 -> If Action Subsystem1/Action
  If/3 -> If Action Subsystem2/Action
  If/4 -> If Action Subsystem3/Action
  Constant2/1 -> If Action Subsystem2/1(In1)
  Constant1/1 -> If Action Subsystem1/1(In1)
  Constant3/1 -> If Action Subsystem3/1(In1)
  Subsystem2/1(Out1) -> If/1
  Subsystem3/1(Out1) -> If/2
  Subsystem4/1(Out1) -> If/3
  Subsystem5/1(Out1) -> If/4
  Subsystem6/1(Out1) -> Sum/7
  If Action Subsystem/1(Out1) -> Sum/3
  If Action Subsystem1/1(Out1) -> Sum/4
  If Action Subsystem2/1(Out1) -> Sum/5
  If Action Subsystem3/1(Out1) -> Sum/6

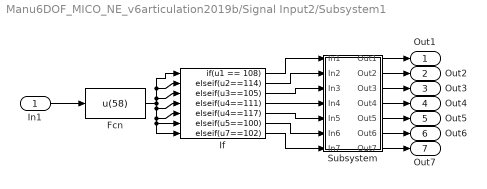
== system Manu6DOF_MICO_NE_v6articulation2019b/Signal Input2/Subsystem1 ==
  In1 : Inport
  Fcn : Fcn  Expr=u(58)
  If : If  NumInputs=7  IfExpression=u1 == 108  ElseIfExpressions=u2==114,u3==105,u4==111,u4==117,u5==100,u7==102  ShowElse=off
  Subsystem : Subsystem
  Out1 : Outport
  Out2 : Outport  Port=2
  Out3 : Outport  Port=3
  Out4 : Outport  Port=4
  Out5 : Outport  Port=5
  Out6 : Outport  Port=6
  Out7 : Outport  Port=7
  wires:
  If/6 -> Subsystem/6(In6)
  If/2 -> Subsystem/2(In2)
  If/4 -> Subsystem/4(In4)
  If/7 -> Subsystem/7(In7)
  If/3 -> Subsystem/3(In3)
  Fcn/1 -> If/1, If/2, If/3, If/7, If/6, If/5, If/4
  If/1 -> Subsystem/1(In1)
  If/5 -> Subsystem/5(In5)
  Subsystem/1(Out1) -> Out1/1
  Subsystem/2(Out2) -> Out2/1
  Subsystem/3(Out3) -> Out3/1
  In1/1 -> Fcn/1
  Subsystem/6(Out6) -> Out6/1
  Subsystem/5(Out5) -> Out5/1
  Subsystem/4(Out4) -> Out4/1
  Subsystem/7(Out7) -> Out7/1

== system Manu6DOF_MICO_NE_v6articulation2019b/Signal Input2/Iterator Input/If Action Subsystem ==
  In1 : Inport
  Action Port : ActionPort  InitializeStates=reset  ActionPortLabel=if(u1 == 3)
  Out1 : Outport  OutputWhenDisabled=reset  InitialOutput=[0]
  wires:
  In1/1 -> Out1/1

== system Manu6DOF_MICO_NE_v6articulation2019b/Signal Input2/Iterator Input/If Action Subsystem1 ==
  In1 : Inport
  Action Port : ActionPort  InitializeStates=reset  ActionPortLabel=elseif(u2==6)
  Out1 : Outport  OutputWhenDisabled=reset  InitialOutput=[0]
  wires:
  In1/1 -> Out1/1

== system Manu6DOF_MICO_NE_v6articulation2019b/Signal Input2/Iterator Input/If Action Subsystem2 ==
  In1 : Inport
  Action Port : ActionPort  InitializeStates=reset  ActionPortLabel=elseif(u3==2)
  Out1 : Outport  OutputWhenDisabled=reset  InitialOutput=[0]
  wires:
  In1/1 -> Out1/1

== system Manu6DOF_MICO_NE_v6articulation2019b/Signal Input2/Iterator Input/If Action Subsystem3 ==
  In1 : Inport
  Action Port : ActionPort  InitializeStates=reset  ActionPortLabel=elseif(u4==5)
  Out1 : Outport  OutputWhenDisabled=reset  InitialOutput=[0]
  wires:
  In1/1 -> Out1/1

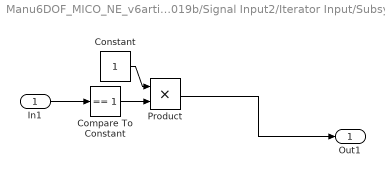
== system Manu6DOF_MICO_NE_v6articulation2019b/Signal Input2/Iterator Input/Subsystem ==
  In1 : Inport
  Compare To Constant : simulink/Logic and Bit Operations/Compare To Constant  relop===  const=1  OutDataTypeStr=boolean
  Constant : Constant
  Product : Product
  Out1 : Outport
  wires:
  Constant/1 -> Product/1
  Compare To Constant/1 -> Product/2
  In1/1 -> Compare To Constant/1
  Product/1 -> Out1/1

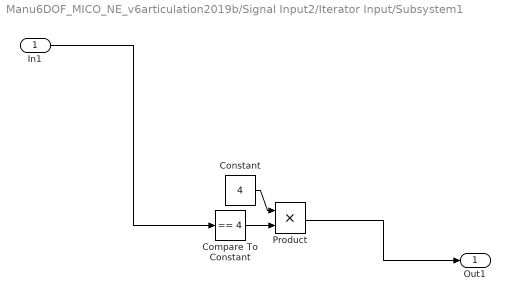
== system Manu6DOF_MICO_NE_v6articulation2019b/Signal Input2/Iterator Input/Subsystem1 ==
  In1 : Inport
  Compare To Constant : simulink/Logic and Bit Operations/Compare To Constant  relop===  const=4  OutDataTypeStr=boolean
  Constant : Constant  Value=4
  Product : Product
  Out1 : Outport
  wires:
  Product/1 -> Out1/1
  In1/1 -> Compare To Constant/1
  Compare To Constant/1 -> Product/2
  Constant/1 -> Product/1

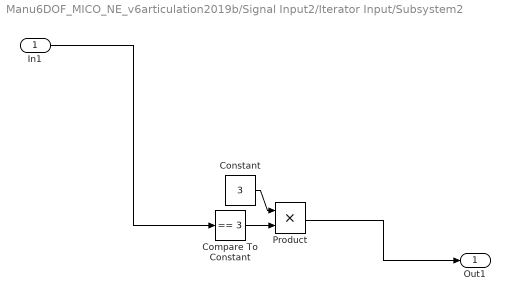
== system Manu6DOF_MICO_NE_v6articulation2019b/Signal Input2/Iterator Input/Subsystem2 ==
  In1 : Inport
  Compare To Constant : simulink/Logic and Bit Operations/Compare To Constant  relop===  const=3  OutDataTypeStr=boolean
  Constant : Constant  Value=3
  Product : Product
  Out1 : Outport
  wires:
  Constant/1 -> Product/1
  Compare To Constant/1 -> Product/2
  In1/1 -> Compare To Constant/1
  Product/1 -> Out1/1

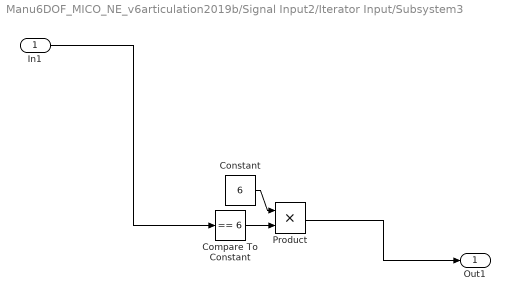
== system Manu6DOF_MICO_NE_v6articulation2019b/Signal Input2/Iterator Input/Subsystem3 ==
  In1 : Inport
  Compare To Constant : simulink/Logic and Bit Operations/Compare To Constant  relop===  const=6  OutDataTypeStr=boolean
  Constant : Constant  Value=6
  Product : Product
  Out1 : Outport
  wires:
  Product/1 -> Out1/1
  In1/1 -> Compare To Constant/1
  Compare To Constant/1 -> Product/2
  Constant/1 -> Product/1

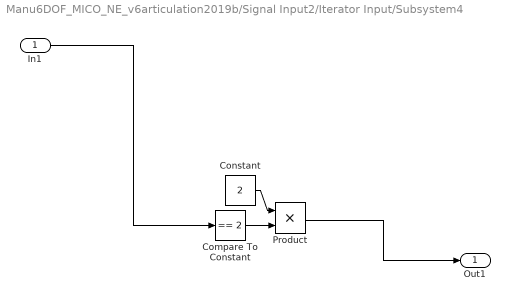
== system Manu6DOF_MICO_NE_v6articulation2019b/Signal Input2/Iterator Input/Subsystem4 ==
  In1 : Inport
  Compare To Constant : simulink/Logic and Bit Operations/Compare To Constant  relop===  const=2  OutDataTypeStr=boolean
  Constant : Constant  Value=2
  Product : Product
  Out1 : Outport
  wires:
  Constant/1 -> Product/1
  Compare To Constant/1 -> Product/2
  In1/1 -> Compare To Constant/1
  Product/1 -> Out1/1

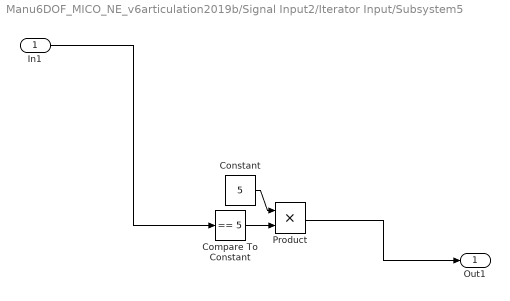
== system Manu6DOF_MICO_NE_v6articulation2019b/Signal Input2/Iterator Input/Subsystem5 ==
  In1 : Inport
  Compare To Constant : simulink/Logic and Bit Operations/Compare To Constant  relop===  const=5  OutDataTypeStr=boolean
  Constant : Constant  Value=5
  Product : Product
  Out1 : Outport
  wires:
  Product/1 -> Out1/1
  In1/1 -> Compare To Constant/1
  Compare To Constant/1 -> Product/2
  Constant/1 -> Product/1

== system Manu6DOF_MICO_NE_v6articulation2019b/Signal Input2/Iterator Input/Subsystem6 ==
  In1 : Inport
  Compare To Constant : simulink/Logic and Bit Operations/Compare To Constant  relop===  const=0  OutDataTypeStr=boolean
  Constant : Constant  Value=0
  Product : Product
  Out1 : Outport
  wires:
  Constant/1 -> Product/1
  Compare To Constant/1 -> Product/2
  In1/1 -> Compare To Constant/1
  Product/1 -> Out1/1

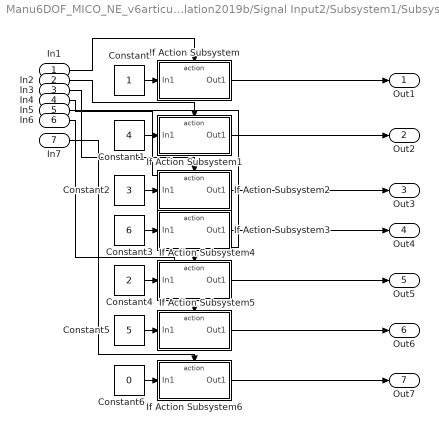
== system Manu6DOF_MICO_NE_v6articulation2019b/Signal Input2/Subsystem1/Subsystem ==
  In1 : Inport
  In2 : Inport  Port=2
  In3 : Inport  Port=3
  In4 : Inport  Port=4
  In5 : Inport  Port=5
  In6 : Inport  Port=6
  In7 : Inport  Port=7
  Constant : Constant
  Constant1 : Constant  Value=4
  Constant2 : Constant  Value=3
  Constant3 : Constant  Value=6
  Constant4 : Constant  Value=2
  Constant5 : Constant  Value=5
  Constant6 : Constant  Value=0
  If Action Subsystem : Subsystem  TreatAsAtomicUnit=on
  If Action Subsystem1 : Subsystem  TreatAsAtomicUnit=on
  If Action Subsystem2 : Subsystem  TreatAsAtomicUnit=on
  If Action Subsystem3 : Subsystem  TreatAsAtomicUnit=on
  If Action Subsystem4 : Subsystem  TreatAsAtomicUnit=on
  If Action Subsystem5 : Subsystem  TreatAsAtomicUnit=on
  If Action Subsystem6 : Subsystem  TreatAsAtomicUnit=on
  Out1 : Outport
  Out2 : Outport  Port=2
  Out3 : Outport  Port=3
  Out4 : Outport  Port=4
  Out5 : Outport  Port=5
  Out6 : Outport  Port=6
  Out7 : Outport  Port=7
  wires:
  Constant/1 -> If Action Subsystem/1(In1)
  In2/1 -> If Action Subsystem1/Action
  Constant2/1 -> If Action Subsystem2/1(In1)
  In4/1 -> If Action Subsystem3/Action
  Constant5/1 -> If Action Subsystem5/1(In1)
  Constant1/1 -> If Action Subsystem1/1(In1)
  In3/1 -> If Action Subsystem2/Action
  If Action Subsystem/1(Out1) -> Out1/1
  Constant3/1 -> If Action Subsystem3/1(In1)
  In1/1 -> If Action Subsystem/Action
  Constant4/1 -> If Action Subsystem4/1(In1)
  In6/1 -> If Action Subsystem5/Action
  If Action Subsystem2/1(Out1) -> Out3/1
  If Action Subsystem4/1(Out1) -> Out5/1
  If Action Subsystem3/1(Out1) -> Out4/1
  In5/1 -> If Action Subsystem4/Action
  If Action Subsystem5/1(Out1) -> Out6/1
  If Action Subsystem1/1(Out1) -> Out2/1
  Constant6/1 -> If Action Subsystem6/1(In1)
  In7/1 -> If Action Subsystem6/Action
  If Action Subsystem6/1(Out1) -> Out7/1

== system Manu6DOF_MICO_NE_v6articulation2019b/Signal Input2/Subsystem1/Subsystem/If Action Subsystem ==
  In1 : Inport
  Action Port : ActionPort  InitializeStates=reset  ActionPortLabel=if(u1 == 108)
  Out1 : Outport  OutputWhenDisabled=reset  InitialOutput=[0]
  wires:
  In1/1 -> Out1/1

== system Manu6DOF_MICO_NE_v6articulation2019b/Signal Input2/Subsystem1/Subsystem/If Action Subsystem1 ==
  In1 : Inport
  Action Port : ActionPort  InitializeStates=reset  ActionPortLabel=elseif(u2==114)
  Out1 : Outport  OutputWhenDisabled=reset  InitialOutput=[0]
  wires:
  In1/1 -> Out1/1

== system Manu6DOF_MICO_NE_v6articulation2019b/Signal Input2/Subsystem1/Subsystem/If Action Subsystem2 ==
  In1 : Inport
  Action Port : ActionPort  InitializeStates=reset  ActionPortLabel=elseif(u3==105)
  Out1 : Outport  OutputWhenDisabled=reset  InitialOutput=[0]
  wires:
  In1/1 -> Out1/1

== system Manu6DOF_MICO_NE_v6articulation2019b/Signal Input2/Subsystem1/Subsystem/If Action Subsystem3 ==
  In1 : Inport
  Action Port : ActionPort  InitializeStates=reset  ActionPortLabel=elseif(u4==111)
  Out1 : Outport  OutputWhenDisabled=reset  InitialOutput=[0]
  wires:
  In1/1 -> Out1/1

== system Manu6DOF_MICO_NE_v6articulation2019b/Signal Input2/Subsystem1/Subsystem/If Action Subsystem4 ==
  In1 : Inport
  Action Port : ActionPort  InitializeStates=reset  ActionPortLabel=elseif(u4==117)
  Out1 : Outport  OutputWhenDisabled=reset  InitialOutput=[0]
  wires:
  In1/1 -> Out1/1

== system Manu6DOF_MICO_NE_v6articulation2019b/Signal Input2/Subsystem1/Subsystem/If Action Subsystem5 ==
  In1 : Inport
  Action Port : ActionPort  InitializeStates=reset  ActionPortLabel=elseif(u5==100)
  Out1 : Outport  OutputWhenDisabled=reset  InitialOutput=[0]
  wires:
  In1/1 -> Out1/1

== system Manu6DOF_MICO_NE_v6articulation2019b/Signal Input2/Subsystem1/Subsystem/If Action Subsystem6 ==
  In1 : Inport
  Action Port : ActionPort  InitializeStates=reset  ActionPortLabel=elseif(u7==102)
  Out1 : Outport  OutputWhenDisabled=reset  InitialOutput=[0]
  wires:
  In1/1 -> Out1/1
